simulink model "Hinf"  (R2021b)
settings: Solver=VariableStepAuto  StartTime=0.0  StopTime=10.0  RelTol=1e-3
values from neighbouring files (symbols this model uses):
  A = [[0 1 0] ... (first row only)    [Hinfmodel.m]    (also in LQGModel.m = [[0 1]; Model.m = [[0 1]; NewModel.m; RunFromMatlab.m = [[0 1])
  B = [[0] ... (first row only)    [Hinfmodel.m]    (also in LQGModel.m = [-0.07528015464; Model.m = [-1; NewModel.m; RunFromMatlab.m = [-0.07528015464)
  C = [[1/40.33*0.9 0 0] ... (first row only)    [Hinfmodel.m]    (also in LQGModel.m = [[0.6 0]; Model.m = [[1 0]; NewModel.m; RunFromMatlab.m = [[0.5 0])
  D = [0;0;0]    [Hinfmodel.m]    (also in LQGModel.m = [0; Model.m = [0; NewModel.m; RunFromMatlab.m = [0)
  K = [-0.3972  -0.8279]    [DampingExperiments.m]    (also in LQGModel.m = place(A,B,[-0.2 + 0.1i -0.2-0.1i]); Model.m = 0.0284001563974)
undefined symbols (not defined in the file or in its folder): Kinf
settings Model: Creator=wsboer  LastModifiedBy=wsboer

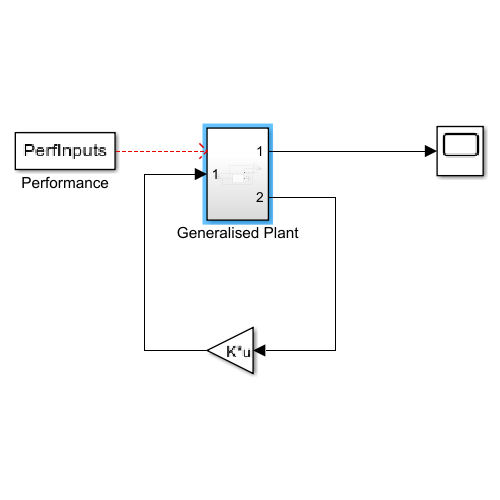
[thumbnail: Simulink's stored preview of the top-level diagram]
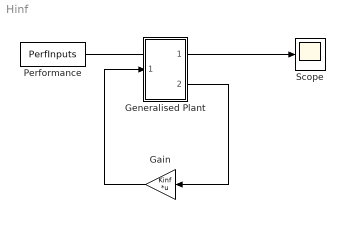
== system Hinf ==
  Gain : Gain  Gain=Kinf  Multiplication=Matrix(K*u)
  Generalised Plant : Subsystem
  Performance : FromWorkspace  VariableName=PerfInputs
  Scope : Scope
  wires:
  Performance/1 -> ?
  Gain/1 -> Generalised Plant/1(In2)
  Generalised Plant/1(Out1) -> Scope/1
  Generalised Plant/2(Out2) -> Gain/1

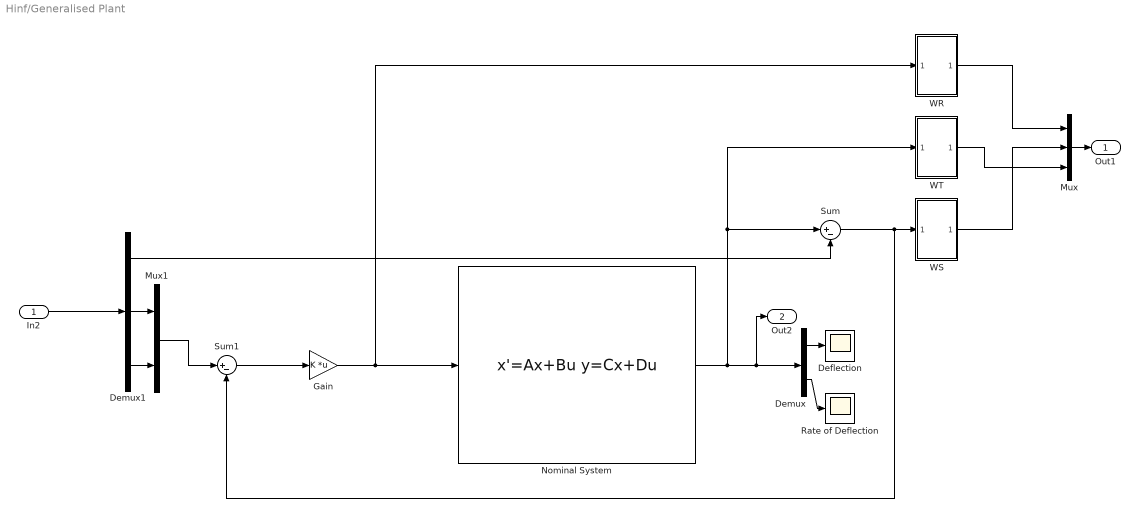
== system Hinf/Generalised Plant ==
  In2 : Inport
  Deflection : Scope
  Demux : Demux  Outputs=2
  Demux1 : Demux  Outputs=3
  Gain : Gain  Gain=K  Multiplication=Matrix(K*u)
  Mux : Mux  Inputs=3
  Mux1 : Mux  Inputs=2
  Nominal System : StateSpace  A=A  B=B  C=C  D=D  InitialCondition=0  ParameterTunability=Unconstrained  ContinuousStateAttributes='sys.StateName'
  Rate of Deflection : Scope
  Sum : Sum  Inputs=|+-
  Sum1 : Sum  Inputs=|+-
  WR : Subsystem
  WS : Subsystem
  WT : Subsystem
  Out1 : Outport
  Out2 : Outport  Port=2
  wires:
  WR/1(Out1) -> Mux/1
  Nominal System/1 -> Sum/1, WT/1(In1), Out2/1, Demux/1
  Gain/1 -> WR/1(In1), Nominal System/1
  Demux/2 -> Rate of Deflection/1
  WT/1(Out1) -> Mux/3
  Demux/1 -> Deflection/1
  Sum1/1 -> Gain/1
  WS/1(Out1) -> Mux/2
  Sum/1 -> Sum1/2, WS/1(In1)
  Mux/1 -> Out1/1
  Demux1/1 -> Sum/2
  In2/1 -> Demux1/1
  Demux1/3 -> Mux1/2
  Demux1/2 -> Mux1/1
  Mux1/1 -> Sum1/1

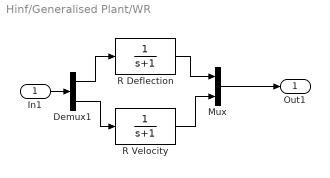
== system Hinf/Generalised Plant/WR ==
  In1 : Inport
  Demux1 : Demux  Outputs=2
  Mux : Mux  Inputs=2
  R Deflection : TransferFcn  Denominator=[1 1]
  R Velocity : TransferFcn  Denominator=[1 1]
  Out1 : Outport
  wires:
  R Deflection/1 -> Mux/1
  R Velocity/1 -> Mux/2
  Demux1/1 -> R Deflection/1
  Demux1/2 -> R Velocity/1
  Mux/1 -> Out1/1
  In1/1 -> Demux1/1

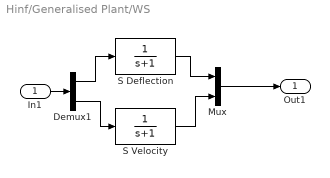
== system Hinf/Generalised Plant/WS ==
  In1 : Inport
  Demux1 : Demux  Outputs=2
  Mux : Mux  Inputs=2
  S Deflection : TransferFcn  Denominator=[1 1]
  S Velocity : TransferFcn  Denominator=[1 1]
  Out1 : Outport
  wires:
  S Deflection/1 -> Mux/1
  S Velocity/1 -> Mux/2
  Demux1/1 -> S Deflection/1
  Demux1/2 -> S Velocity/1
  Mux/1 -> Out1/1
  In1/1 -> Demux1/1

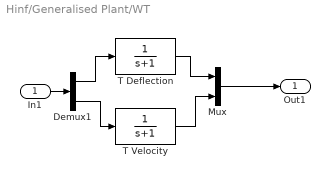
== system Hinf/Generalised Plant/WT ==
  In1 : Inport
  Demux1 : Demux  Outputs=2
  Mux : Mux  Inputs=2
  T Deflection : TransferFcn  Denominator=[1 1]
  T Velocity : TransferFcn  Denominator=[1 1]
  Out1 : Outport
  wires:
  T Deflection/1 -> Mux/1
  T Velocity/1 -> Mux/2
  Demux1/1 -> T Deflection/1
  Demux1/2 -> T Velocity/1
  Mux/1 -> Out1/1
  In1/1 -> Demux1/1
